simulink model "FUZZY_tsc_neurospora_model_leloup_za_sliko"  (R2015a)
settings: Solver=ode4  StartTime=0.0  StopTime=72  FixedStep=0.01  RelTol=1e-3
values from neighbouring files (symbols this model uses):
  k_1 = 0.5    [ALL_neurospora_init.m]    (also in FUZZY_deg_neurospora_init.m; FUZZY_tsc_neurospora_init.m; FUZZY_tsc_tsl_neurospora_init.m; FUZZY_tsl_neurospora_init.m)
  k_2 = 0.6    [ALL_neurospora_init.m]    (also in FUZZY_deg_neurospora_init.m; FUZZY_tsc_neurospora_init.m; FUZZY_tsc_tsl_neurospora_init.m; FUZZY_tsl_neurospora_init.m)
  K_d = 0.13    [ALL_neurospora_init.m]    (also in FUZZY_deg_neurospora_init.m; FUZZY_tsc_neurospora_init.m; FUZZY_tsc_tsl_neurospora_init.m; FUZZY_tsl_neurospora_init.m)
  K_m = 0.5    [ALL_neurospora_init.m]    (also in FUZZY_deg_neurospora_init.m; FUZZY_tsc_neurospora_init.m; FUZZY_tsc_tsl_neurospora_init.m; FUZZY_tsl_neurospora_init.m)
  k_s = 0.5    [ALL_neurospora_init.m]    (also in FUZZY_deg_neurospora_init.m; FUZZY_tsc_neurospora_init.m; FUZZY_tsc_tsl_neurospora_init.m; FUZZY_tsl_neurospora_init.m)
  v_d = 1.4    [ALL_neurospora_init.m]    (also in FUZZY_deg_neurospora_init.m; FUZZY_tsc_neurospora_init.m; FUZZY_tsc_tsl_neurospora_init.m; FUZZY_tsl_neurospora_init.m)
  v_m = 0.505    [ALL_neurospora_init.m]    (also in FUZZY_deg_neurospora_init.m; FUZZY_tsc_neurospora_init.m; FUZZY_tsc_tsl_neurospora_init.m; FUZZY_tsl_neurospora_init.m)
libraries: fuzblock x1
settings Model: Creator=jureb  LastModifiedBy=jure

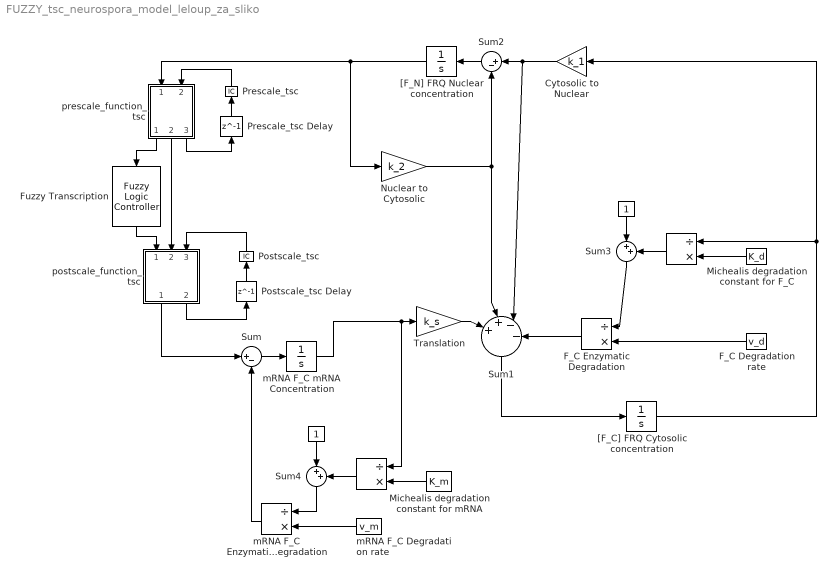
== system FUZZY_tsc_neurospora_model_leloup_za_sliko ==
  " " : Product  Inputs=/*
  " " : Constant
  " " : Constant
  " " : Product  Inputs=/*
  Cytosolic to Nuclear : Gain  Gain=k_1
  F_C Degradation rate : Constant  Value=v_d
  F_C Enzymatic Degradation : Product  Inputs=/*
  Fuzzy Transcription : fuzblock/Fuzzy Logic  Controller  fis=tsc
  Michealis degradation constant for F_C : Constant  Value=K_d
  Michealis degradation constant for mRNA : Constant  Value=K_m
  Nuclear to Cytosolic : Gain  Gain=k_2
  Postscale_tsc : InitialCondition  Value=1.3
  Postscale_tsc Delay : Delay  DelayLength=1  InitialCondition=1
  Prescale_tsc : InitialCondition  Value=5
  Prescale_tsc Delay : Delay  DelayLength=1  InitialCondition=1  UseCircularBuffer=on
  Sum : Sum  Inputs=|+-
  Sum1 : Sum  Inputs=|+|+|-|-
  Sum2 : Sum  Inputs=|+-
  Sum3 : Sum  Inputs=|++
  Sum4 : Sum  Inputs=|++
  Translation : Gain  Gain=k_s
  "[F_C] FRQ Cytosolic concentration " : Integrator  InitialCondition=1
  "[F_N] FRQ Nuclear concentration" : Integrator  InitialCondition=1
  mRNA F_C Degradation rate : Constant  Value=v_m
  mRNA F_C Enzymatic Degradation : Product  Inputs=/*
  mRNA F_C mRNA Concentration : Integrator  InitialCondition=1
  postscale_function_tsc : MATLAB Function  TreatAsAtomicUnit=on
  prescale_function_tsc : MATLAB Function  TreatAsAtomicUnit=on
  wires:
  Sum/1 -> mRNA F_C mRNA Concentration/1
  mRNA F_C mRNA Concentration/1 -> " "/1, Translation/1
  mRNA F_C Enzymatic Degradation/1 -> Sum/2
  "[F_N] FRQ Nuclear concentration"/1 -> prescale_function_tsc/1(input), Nuclear to Cytosolic/1
  Sum1/1 -> "[F_C] FRQ Cytosolic concentration "/1
  Cytosolic to Nuclear/1 -> Sum1/3, Sum2/1
  Sum2/1 -> "[F_N] FRQ Nuclear concentration"/1
  Nuclear to Cytosolic/1 -> Sum1/2, Sum2/2
  mRNA F_C Degradation rate/1 -> mRNA F_C Enzymatic Degradation/2
  " "/1 -> Sum4/1
  " "/1 -> Sum4/2
  Michealis degradation constant for mRNA/1 -> " "/2
  Sum4/1 -> mRNA F_C Enzymatic Degradation/1
  "[F_C] FRQ Cytosolic concentration "/1 -> Cytosolic to Nuclear/1, " "/1
  F_C Enzymatic Degradation/1 -> Sum1/4
  F_C Degradation rate/1 -> F_C Enzymatic Degradation/2
  " "/1 -> Sum3/1
  " "/1 -> Sum3/2
  Michealis degradation constant for F_C/1 -> " "/2
  Sum3/1 -> F_C Enzymatic Degradation/1
  Translation/1 -> Sum1/1
  prescale_function_tsc/3(prescale_out) -> Prescale_tsc Delay/1
  Prescale_tsc/1 -> prescale_function_tsc/2(prescale_in)
  Postscale_tsc/1 -> postscale_function_tsc/3(postscale_in)
  postscale_function_tsc/2(postscale_out) -> Postscale_tsc Delay/1
  Prescale_tsc Delay/1 -> Prescale_tsc/1
  Postscale_tsc Delay/1 -> Postscale_tsc/1
  prescale_function_tsc/1(input_prescaled) -> Fuzzy Transcription/1
  postscale_function_tsc/1(output_postscaled) -> Sum/1
  Fuzzy Transcription/1 -> postscale_function_tsc/1(output)
  prescale_function_tsc/2(prescale_changed) -> postscale_function_tsc/2(prescale_changed)

== matlab function FUZZY_tsc_neurospora_model_leloup_za_sliko/prescale_function_tsc ==
  data: input input; input_prescaled output; prescale_changed output; prescale_in input; prescale_out output
function [input_prescaled, prescale_changed, prescale_out] = prescale(input, prescale_in)

prescale_out = prescale_in;
multiplier = 1.01;
prescale_changed = 0;

if (input >= 0.9*prescale_in)
    prescale_out = prescale_in*multiplier;
    prescale_changed = 1;
end

input_prescaled = input/prescale_out;

== matlab function FUZZY_tsc_neurospora_model_leloup_za_sliko/postscale_function_tsc ==
  data: output input; prescale_changed input; output_postscaled output; postscale_in input; postscale_out output
function [output_postscaled, postscale_out] = postscale(output, prescale_changed, postscale_in)

postscale_out = postscale_in;
multiplier = 1.01;

if (prescale_changed == 1)
    postscale_out = postscale_out*multiplier;
end

output_postscaled = output*postscale_out;
